simulink model "sl_arm_ibvs2"  (R2015b)
settings: Solver=ode45  StartTime=0.0  StopTime=20.0  RelTol=1e-3
InitFcn:
  | mdl_puma560
  | camera = CentralCamera('default');
  | P = mkgrid(2, 0.5, troty(pi/2)*transl(0,0,2.5));
  | q0 = [0 pi/4 pi 0 pi/4 -pi/4]';
libraries: roblocks x9
settings Model: ExtModeTrigMode=oneshot  ExtModeArmWhenConnect=off  Creator=pic  LastModifiedBy=corkep
settings DataIOCC: LimitDataPoints=off  SaveFormat=StructureWithTime  SignalLoggingSaveFormat=ModelDataLogs  ReturnWorkspaceOutputs=on
settings OptimizationCC: BlockReduction=off  BooleanDataType=off  ExpressionDepthLimit=2147483647  InitFltsAndDblsToZero=on
settings DebuggingCC: SaveWithParameterizedLinksMsg=none  UnderspecifiedInitializationDetection=Classic  MergeDetectMultiDrivingBlocksExec=none  SignalResolutionControl=TryResolveAllWithWarning  MultiTaskDSMMsg=warning  MultiTaskCondExecSysMsg=none  FcnCallInpInsideContextMsg=UseLocalSettings  StateNameClashWarn=warning
settings HardwareCC: ProdBitPerPointer=32  ProdLargestAtomicFloat=None  ProdIntDivRoundTo=Undefined  ProdEndianess=Unspecified  ProdWordSize=32  ProdHWDeviceType=32-bit Generic  TargetUnknown=on
settings GRTTargetCC: ModelReferenceCompliant=off  CompOptLevelCompliant=off  GeneratePreprocessorConditionals=Disable all  CombineOutputUpdateFcns=off  MatFileLogging=off  GRTInterface=on
settings ConfigComp: CovModelRefEnable=Off  CovSFcnEnable=off

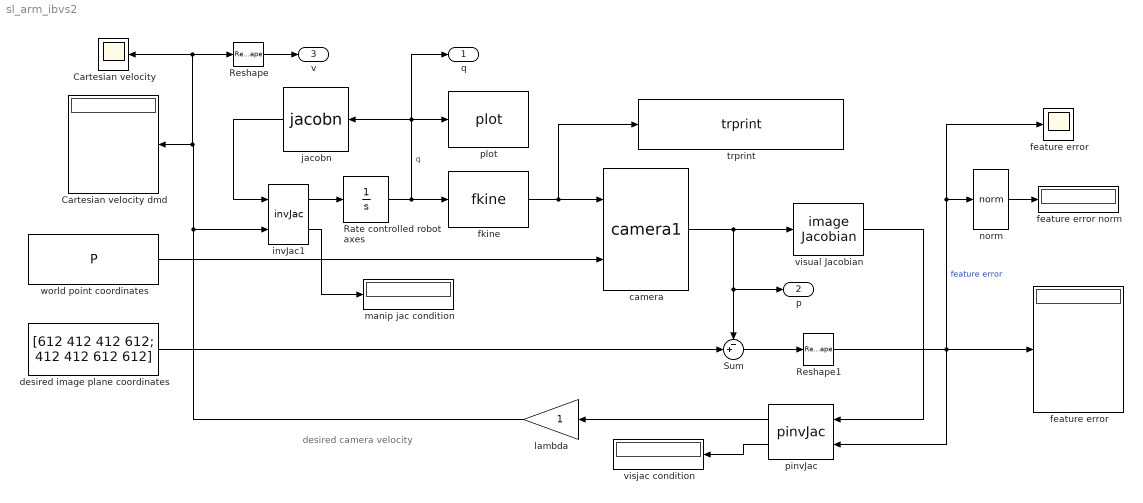
== system sl_arm_ibvs2 ==
  note: desired camera velocity
  Cartesian velocity : Scope
  Cartesian velocity dmd : Display
      settings: Format=bank
  Rate controlled robot axes : Integrator  InitialCondition=q0
  Reshape : Reshape  OutputDimensions=6
  Reshape1 : Reshape  OutputDimensions=6
  Sum : Sum  Inputs=-+|  SaturateOnIntegerOverflow=on  InputSameDT=on  OutDataTypeStr=Inherit: Same as first input
  camera : roblocks/Vision/camera1  cam=cam
  desired image plane coordinates : Constant  Value=[612 412 412 612; 412 412 612 612]  VectorParams1D=off
  feature error : Display
      settings: Format=bank
  feature error norm : Display
  "feature error " : Scope
  fkine : roblocks/Arm/fkine  robot=p560
  invJac1 : roblocks/Toolbox/invJac
  jacobn : roblocks/Arm/jacobn  robot=p560
  lambda : Gain  SaturateOnIntegerOverflow=on  OutDataTypeStr=Inherit: Same as input  ParamDataTypeStr=Inherit: Same as input
  manip jac condition : Display
  norm : roblocks/Toolbox/norm  SystemSampleTime=-1
  pinvJac : roblocks/Toolbox/pinvJac
  plot : roblocks/Arm/plot  robot=p560  fps=25  holdplot=on
  trprint : roblocks/Toolbox/trprint  options={'bingo'}
      link override S-Function: Parameters=options
  visjac condition : Display
  visual Jacobian : roblocks/Vision/image Jacobian  cam=cam  z=3
  world point coordinates : Constant  Value=P  VectorParams1D=off
  q : Outport
  p : Outport  Port=2
  v : Outport  Port=3
  wires:
  Rate controlled robot axes/1 -> jacobn/1, plot/1, q/1, fkine/1  "q"
  jacobn/1 -> invJac1/1
  invJac1/1 -> Rate controlled robot axes/1
  invJac1/2 -> manip jac condition/1
  Sum/1 -> Reshape1/1
  desired image plane coordinates/1 -> Sum/2
  Reshape1/1 -> feature error/1, pinvJac/2, "feature error "/1, norm/1  "feature error"
  pinvJac/2 -> visjac condition/1
  pinvJac/1 -> lambda/1
  fkine/1 -> trprint/1, camera/1
  visual Jacobian/1 -> pinvJac/1
  lambda/1 -> Reshape/1, Cartesian velocity/1, Cartesian velocity dmd/1, invJac1/2
  Reshape/1 -> v/1
  camera/1 -> Sum/1, p/1, visual Jacobian/1
  world point coordinates/1 -> camera/2
  norm/1 -> feature error norm/1
